simulink model "MPC_regul_linear"  (R2017a)
settings: Solver=VariableStepAuto  StartTime=0.0  StopTime=100  RelTol=1e-3
undefined symbols (not defined in the file): Asystem, Bsystem, Ts
settings Model: Creator=sverreknutsen  LastModifiedBy=sverreknutsen

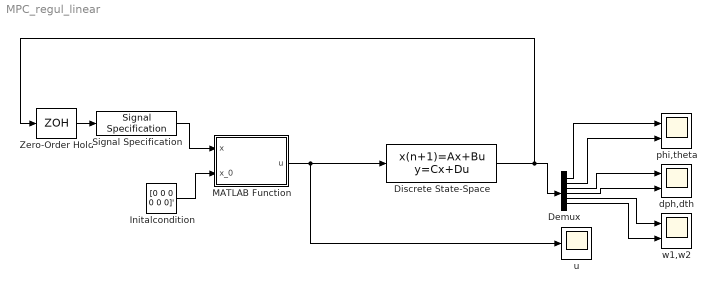
== system MPC_regul_linear ==
  Demux : Demux  Outputs=6
  Discrete State-Space : DiscreteStateSpace  A=Asystem  B=Bsystem  C=eye(6)  D=zeros(6,2)  X0=[1 1 0 0 0 0]'  SampleTime=Ts
  "Initalcondition " : Constant  Value=[0 0 0 0 0 0]'
  MATLAB Function : MATLAB Function  TreatAsAtomicUnit=on
  Signal Specification : SignalSpecification  Dimensions=[6 1]
  Zero-Order Hold : ZeroOrderHold  SampleTime=Ts
  dph,dth : Scope  NumInputPorts=2
  phi,theta : Scope  NumInputPorts=2
  u : Scope
  w1,w2 : Scope  NumInputPorts=2
  wires:
  Signal Specification/1 -> MATLAB Function/1(x)
  Zero-Order Hold/1 -> Signal Specification/1
  Demux/1 -> phi,theta/1
  "Initalcondition "/1 -> MATLAB Function/2(x_0)
  Demux/3 -> dph,dth/1
  Demux/4 -> dph,dth/2
  Demux/5 -> w1,w2/1
  Demux/6 -> w1,w2/2
  Demux/2 -> phi,theta/2
  Discrete State-Space/1 -> Zero-Order Hold/1, Demux/1
  MATLAB Function/1(u) -> Discrete State-Space/1, u/1

== matlab function MPC_regul_linear/MATLAB Function ==
  data: x input; u output; x_0 input
function u = MPC(x,x_0)
%The MPC solver using CVXgen. 

coder.extrinsic('mycsolve'); %force simulink to accept that mycsolve will acctualy return u in a vector.
u = [0;0]; % pre-define u to be of correct type/size [u] = mycsolve(x);

if(isempty(x)) %initialize
    x=x_0;
    u=mycsolve(x); %solve

else

    u=mycsolve(x); %solve
end
